simulink model "Model_Experiment2_LIFTEC_Paper_Ramon_version16a"  (R2020a)
settings: Solver=VariableStepAuto  StartTime=0.0  StopTime=6000  RelTol=1e-3
values from neighbouring files (symbols this model uses):
  k0_1 = x(1)    [Model_Calibration.m]
  k0_2 = x(2)    [Model_Calibration.m]
undefined symbols (not defined in the file or in its folder): alpha_1, alpha_2, Ccellini2, Ccellini3, Ccellini4, Ccellini5, Chini, Ctankini2, Ctankini3, Ctankini4, Ctankini5, d, D, E0, F, magnitude, N, R, r, S, T, Vcell, Vtank_Anolyte, Vtank_Catholyte
settings Model: Creator=Alejandro  LastModifiedBy=Alejandro
settings OptimizationCC: LifeSpan=inf
settings DebuggingCC: ArithmeticOperatorsInVariantConditions=warning
settings SFSimCC: CustomCodeUndefinedFunction=UseInterfaceOnly
settings CodeAppCC: StateflowObjectComments=on

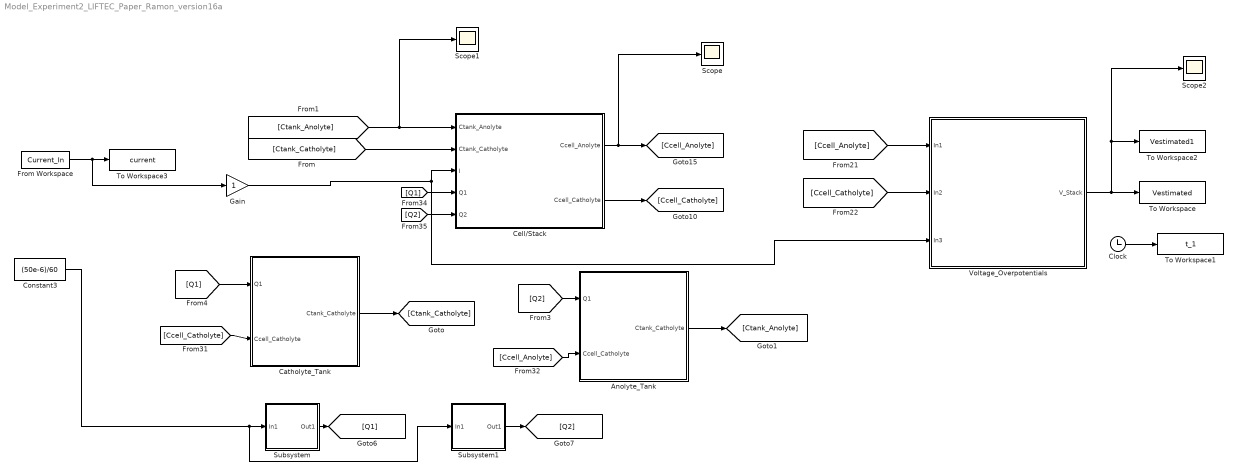
== system Model_Experiment2_LIFTEC_Paper_Ramon_version16a ==
  Anolyte_Tank : Subsystem  mask(Anolyte tank model){}
      mask help: This subsystem defines the model of the anolyte tank of the redox flow batteries..
      mask Help:
      | The parameters of the block consist on:
      | 
      | Vtank_Anolyte: Volume of the anolye tank (m^3)
      | Ctankini2: Initial concentration of V2 in the anolyte tank (mol/m^3)
      | Ctankini3: Initial concentration of V3 in the anolyte tank (mol/m^3)
      mask DialogControl Container4 Prompt: References
      mask DialogControl Control2 Prompt: 1] Tang, A.; McCann, J.; Bao, J.; Skyllas-Kazacos, M. Investigation of the effect of shunt current on battery efficiency and stack temperature in vanadium redox flow battery.
      mask DialogControl Control3 Prompt: https://doi.org/10.1016/j.jpowsour.2013.05.079.
      mask DialogControl Control4 Prompt: 2] Wei, Z.; Xiong, R.; Lim, T.M.; Meng, S.; Skyllas-Kazacos, M.  Online monitoring of state of charge and1010capacity loss for vanadium redox flow battery based on autoregressive exogenous modeling.
      mask DialogControl Control5 Prompt: https://doi.org/10.1016/j.jpowsour.2018.09.028.
      mask Display: image('Anolyte_Tank.JPG')
  Catholyte_Tank : Subsystem  mask(Catholyte tank model){}
      mask help: This subsystem defines the model of the catholyte tank of the redox flow batteries..
      mask Help:
      | The parameters of the block consist on:
      | 
      | Vtank_Catholyte: Volume of the catholyte tank (m^3)
      | Ctankini4: Initial concentration of V4 in the cell (mol/m^3)
      | Ctankini5: Initial concentration of V5 in the cell (mol/m^3)
      mask DialogControl Container4 Prompt: References
      mask DialogControl Control2 Prompt: 1] Tang, A.; McCann, J.; Bao, J.; Skyllas-Kazacos, M. Investigation of the effect of shunt current on battery efficiency and stack temperature in vanadium redox flow battery.
      mask DialogControl Control3 Prompt: https://doi.org/10.1016/j.jpowsour.2013.05.079.
      mask DialogControl Control4 Prompt: 2] Wei, Z.; Xiong, R.; Lim, T.M.; Meng, S.; Skyllas-Kazacos, M.  Online monitoring of state of charge and1010capacity loss for vanadium redox flow battery based on autoregressive exogenous modeling.
      mask DialogControl Control5 Prompt: https://doi.org/10.1016/j.jpowsour.2018.09.028.
      mask Display: image('Catholyte_Tank.JPG')
  Cell/Stack : Subsystem  mask(Cell-Stack model){}
      mask help: This subsystem defines the model of the cell or stack of the redox flow batteries.
      mask Help:
      | The parameters of the block consist on:
      | 
      | N: Number of cells
      | Vcell: Volume of a cell (m^3)
      | S: Electrode surface (m^2)
      | d: Thickness of the membrane (m)
      | Ccellini2: Initial concentration of V2 in the cell (mol/m^3)
      | Ccellini3: Initial concentration of V3 in the cell (mol/m^3)
      | Ccellini4: Initial concentration of V4 in the cell (mol/m^3)
      | Ccellini5: Initial concentration of V5 in the cell (mol/m^3)
      mask DialogControl Container7 Prompt: References
      mask DialogControl Control6 Prompt: 1] Tang, A.; McCann, J.; Bao, J.; Skyllas-Kazacos, M. Investigation of the effect of shunt current on battery efficiency and stack temperature in vanadium redox flow battery.
      mask DialogControl Control7 Prompt: 2] Wei, Z.; Xiong, R.; Lim, T.M.; Meng, S.; Skyllas-Kazacos, M.  Online monitoring of state of charge and1010capacity loss for vanadium redox flow battery based on autoregressive exogenous modeling.
      mask DialogControl Control8 Prompt: https://doi.org/10.1016/j.jpowsour.2018.09.028.
      mask Display: image('Cell.JPG')
  Clock : Clock
  Constant3 : Constant  Value=(50e-6)/60
  From Workspace : FromWorkspace  VariableName=Current_In
  Gain : Gain
  Scope : Scope
  Scope1 : Scope
  Scope2 : Scope
  Subsystem : Subsystem  mask(Pump model){Epump1=1}
      mask help: Model of the pump according to the manufacturer datasheet
      mask Help: Epump: Efficiency of the pump
      mask DialogControl Container4 Prompt: Manufacturer datasheet
      mask DialogControl Control2 Prompt: Model of the pump
      mask Display: image('Pump.JPG')
  Subsystem1 : Subsystem  mask(Pump model){Epump2=1}
      mask help: Model of the pump according to the manufacturer datasheet
      mask Help: Epump2 : Efficiency of the pump
      mask DialogControl Container4 Prompt: Manufacturer datasheet
      mask DialogControl Control2 Prompt: Model of the pump
      mask Display: image('Pump.JPG'); % Use "Edit Image" on toolstrip to change.
  To Workspace : ToWorkspace  VariableName=Vestimated  SampleTime=1.0187
      settings: Save2DSignal=2-D array (concatenate along first dimension)
  To Workspace1 : ToWorkspace  VariableName=t_1  SampleTime=1
      settings: Save2DSignal=2-D array (concatenate along first dimension)
  To Workspace2 : ToWorkspace  VariableName=Vestimated1  SampleTime=1
      settings: Save2DSignal=2-D array (concatenate along first dimension)
  To Workspace3 : ToWorkspace  VariableName=current  SampleTime=1.0
      settings: Save2DSignal=2-D array (concatenate along first dimension)
  Voltage_Overpotentials : Subsystem  mask(Voltage and overpotential){}
      mask help: This block computes the voltage and overpotentials of the cell-stack.
      mask Help:
      | The parameters of the block consist on:
      | 
      | E0: Standard electrode potential (V)
      | r: Ohmic resistance (Ohms)
      | Chini5: Initial concentration of H in the cell (mol/m^3)
      mask DialogControl Container3 Prompt: References
      mask DialogControl Control2 Prompt: (Add text here)
      mask DialogControl Control3 Prompt: (Add text here)
      mask Display: image('Voltage.png')
  wires:
  [Ccell_Catholyte] -> Voltage_Overpotentials/2(In2)
  [Q2] -> Anolyte_Tank/1(Q1)
  [Ccell_Anolyte] -> Anolyte_Tank/2(Ccell_Catholyte)
  [Q1] -> Cell/Stack/4(Q1)
  Catholyte_Tank/1(Ctank_Catholyte) -> [Ctank_Catholyte]
  [Ccell_Catholyte] -> Catholyte_Tank/2(Ccell_Catholyte)
  [Q2] -> Cell/Stack/5(Q2)
  Subsystem/1(Out1) -> [Q1]
  [Ctank_Anolyte] -> Scope1/1, Cell/Stack/1(Ctank_Anolyte)
  [Q1] -> Catholyte_Tank/1(Q1)
  [Ctank_Catholyte] -> Cell/Stack/2(Ctank_Catholyte)
  Subsystem1/1(Out1) -> [Q2]
  From Workspace/1 -> Gain/1, To Workspace3/1
  Constant3/1 -> Subsystem1/1(In1), Subsystem/1(In1)
  Cell/Stack/2(Ccell_Catholyte) -> [Ccell_Catholyte]
  Clock/1 -> To Workspace1/1
  Gain/1 -> Voltage_Overpotentials/3(In3), Cell/Stack/3("I ")
  [Ccell_Anolyte] -> Voltage_Overpotentials/1(In1)
  Anolyte_Tank/1(Ctank_Catholyte) -> [Ctank_Anolyte]
  Voltage_Overpotentials/1(V_Stack) -> Scope2/1, To Workspace2/1, To Workspace/1
  Cell/Stack/1(Ccell_Anolyte) -> Scope/1, [Ccell_Anolyte]

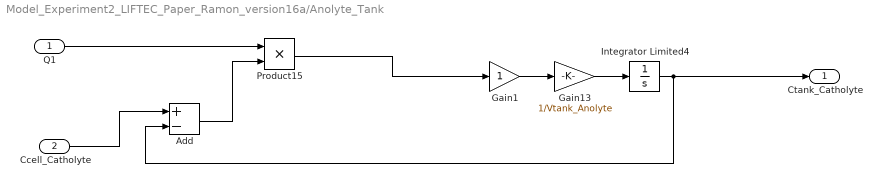
== system Model_Experiment2_LIFTEC_Paper_Ramon_version16a/Anolyte_Tank ==
  Q1 : Inport
  Ccell_Catholyte : Inport  Port=2
  Add : Sum  Inputs=+-
  Gain1 : Gain
  Gain13 : Gain  Gain=1/Vtank_Anolyte
  Integrator Limited4 : Integrator  InitialCondition=[Ctankini2 Ctankini3]  LimitOutput=on  UpperSaturationLimit=400  LowerSaturationLimit=0.001
  Product15 : Product
  Ctank_Catholyte : Outport
  wires:
  Gain13/1 -> Integrator Limited4/1
  Product15/1 -> Gain1/1
  Q1/1 -> Product15/1
  Integrator Limited4/1 -> Ctank_Catholyte/1, Add/2
  Gain1/1 -> Gain13/1
  Ccell_Catholyte/1 -> Add/1
  Add/1 -> Product15/2

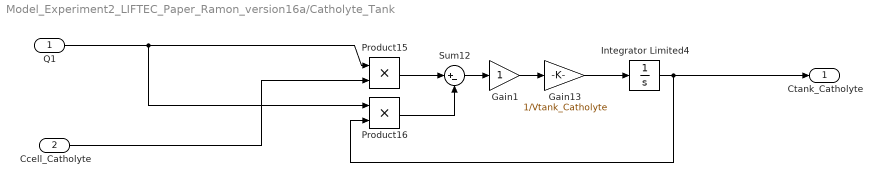
== system Model_Experiment2_LIFTEC_Paper_Ramon_version16a/Catholyte_Tank ==
  Q1 : Inport
  Ccell_Catholyte : Inport  Port=2
  Gain1 : Gain
  Gain13 : Gain  Gain=1/Vtank_Catholyte
  Integrator Limited4 : Integrator  InitialCondition=[Ctankini4 Ctankini5]  LimitOutput=on  UpperSaturationLimit=400  LowerSaturationLimit=0.001
  Product15 : Product
  Product16 : Product
  Sum12 : Sum  Inputs=|+-
  Ctank_Catholyte : Outport
  wires:
  Gain13/1 -> Integrator Limited4/1
  Sum12/1 -> Gain1/1
  Q1/1 -> Product16/1, Product15/1
  Integrator Limited4/1 -> Ctank_Catholyte/1, Product16/2
  Product15/1 -> Sum12/1
  Product16/1 -> Sum12/2
  Ccell_Catholyte/1 -> Product15/2
  Gain1/1 -> Gain13/1

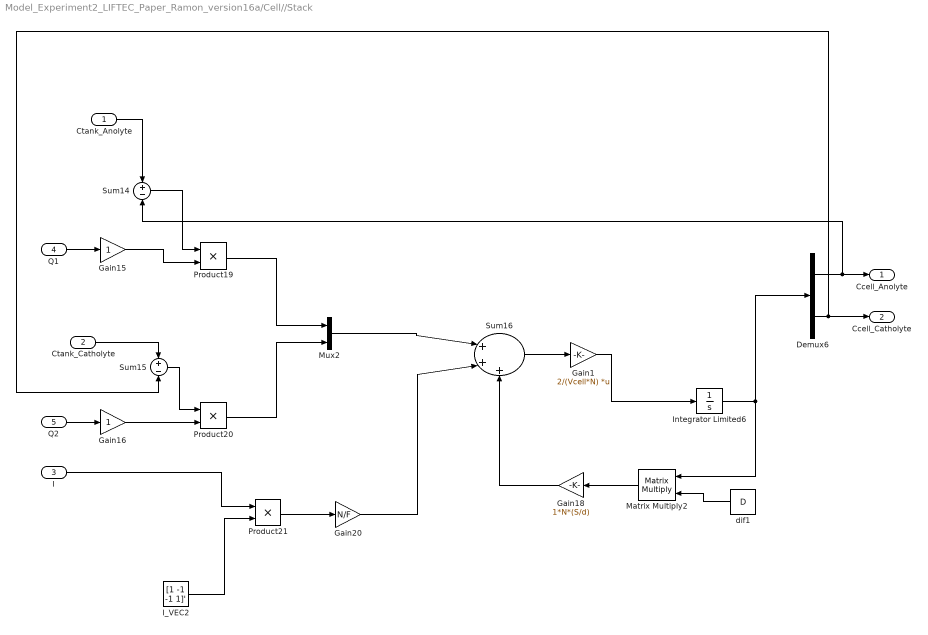
== system Model_Experiment2_LIFTEC_Paper_Ramon_version16a/Cell//Stack ==
  Ctank_Anolyte : Inport
  Ctank_Catholyte : Inport  Port=2
  "I " : Inport  Port=3
  Q1 : Inport  Port=4
  Q2 : Inport  Port=5
  Demux6 : Demux  Outputs=2
  Gain1 : Gain  Gain=2/(Vcell*N)  Multiplication=Matrix(K*u)
  Gain15 : Gain
  Gain16 : Gain
  Gain18 : Gain  Gain=1*N*(S/d)
  Gain20 : Gain  Gain=N/F
  I_VEC2 : Constant  Value=[1 -1 -1 1]'
  Integrator Limited6 : Integrator  InitialCondition=[Ccellini2 Ccellini3 Ccellini4 Ccellini5]  LimitOutput=on  UpperSaturationLimit=400  LowerSaturationLimit=0.001
  Matrix Multiply2 : Product  Multiplication=Matrix(*)
  Mux2 : Mux  Inputs=2
  Product19 : Product
  Product20 : Product
  Product21 : Product
  Sum14 : Sum  Inputs=+-
  Sum15 : Sum  Inputs=+-
  Sum16 : Sum  Inputs=|+++
  dif1 : Constant  Value=D
  Ccell_Anolyte : Outport
  Ccell_Catholyte : Outport  Port=2
  wires:
  Gain18/1 -> Sum16/3
  Ctank_Anolyte/1 -> Sum14/1
  Gain20/1 -> Sum16/2
  "I "/1 -> Product21/1
  Integrator Limited6/1 -> Matrix Multiply2/1, Demux6/1
  Sum16/1 -> Gain1/1
  Gain15/1 -> Product19/2
  Sum14/1 -> Product19/1
  Product21/1 -> Gain20/1
  I_VEC2/1 -> Product21/2
  Product19/1 -> Mux2/1
  Sum15/1 -> Product20/1
  Gain16/1 -> Product20/2
  Q1/1 -> Gain15/1
  Matrix Multiply2/1 -> Gain18/1
  dif1/1 -> Matrix Multiply2/2
  Product20/1 -> Mux2/2
  Ctank_Catholyte/1 -> Sum15/1
  Q2/1 -> Gain16/1
  Mux2/1 -> Sum16/1
  Gain1/1 -> Integrator Limited6/1
  Demux6/1 -> Sum14/2, Ccell_Anolyte/1
  Demux6/2 -> Ccell_Catholyte/1, Sum15/2

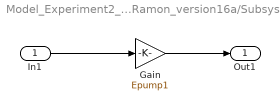
== system Model_Experiment2_LIFTEC_Paper_Ramon_version16a/Subsystem ==
  In1 : Inport
  Gain : Gain  Gain=Epump1
  Out1 : Outport
  wires:
  In1/1 -> Gain/1
  Gain/1 -> Out1/1

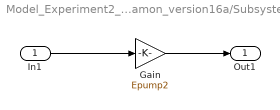
== system Model_Experiment2_LIFTEC_Paper_Ramon_version16a/Subsystem1 ==
  In1 : Inport
  Gain : Gain  Gain=Epump2
  Out1 : Outport
  wires:
  In1/1 -> Gain/1
  Gain/1 -> Out1/1

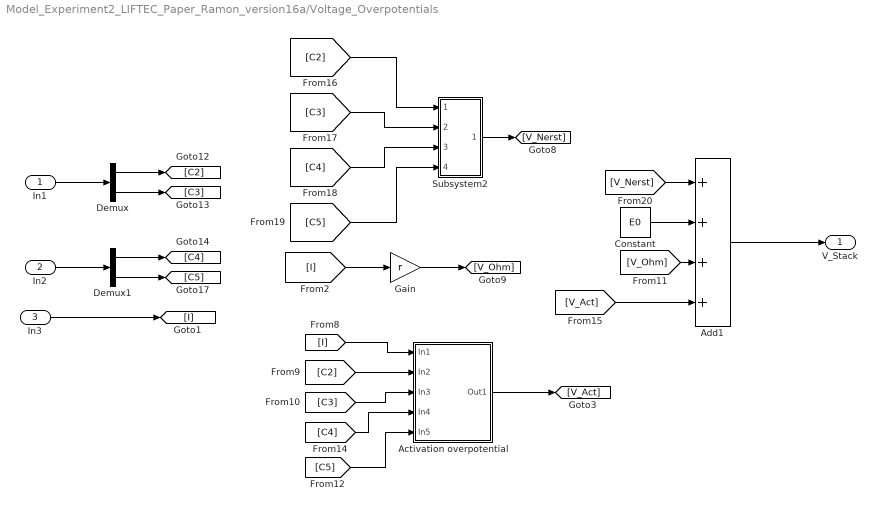
== system Model_Experiment2_LIFTEC_Paper_Ramon_version16a/Voltage_Overpotentials ==
  In1 : Inport
  In2 : Inport  Port=2
  In3 : Inport  Port=3
  Activation overpotential : Subsystem
  Add1 : Sum  Inputs=++++
  Constant : Constant  Value=E0
  Demux : Demux  Outputs=2
  Demux1 : Demux  Outputs=2
  Gain : Gain  Gain=r
  Subsystem2 : Subsystem
  V_Stack : Outport
  wires:
  Add1/1 -> V_Stack/1
  Demux/2 -> [C3]
  Subsystem2/1(Out1) -> [V_Nerst]
  Demux1/2 -> [C5]
  Demux1/1 -> [C4]
  [V_Nerst] -> Add1/1
  Constant/1 -> Add1/2
  Demux/1 -> [C2]
  [V_Ohm] -> Add1/3
  [C2] -> Subsystem2/1(In1)
  [C5] -> Subsystem2/4(In4)
  [C3] -> Subsystem2/2(In2)
  [C4] -> Subsystem2/3(In3)
  In1/1 -> Demux/1
  In2/1 -> Demux1/1
  In3/1 -> [I]
  Gain/1 -> [V_Ohm]
  [I] -> Gain/1
  [I] -> Activation overpotential/1(In1)
  [C2] -> Activation overpotential/2(In2)
  [C3] -> Activation overpotential/3(In3)
  [C4] -> Activation overpotential/4(In4)
  [C5] -> Activation overpotential/5(In5)
  Activation overpotential/1(Out1) -> [V_Act]
  [V_Act] -> Add1/4

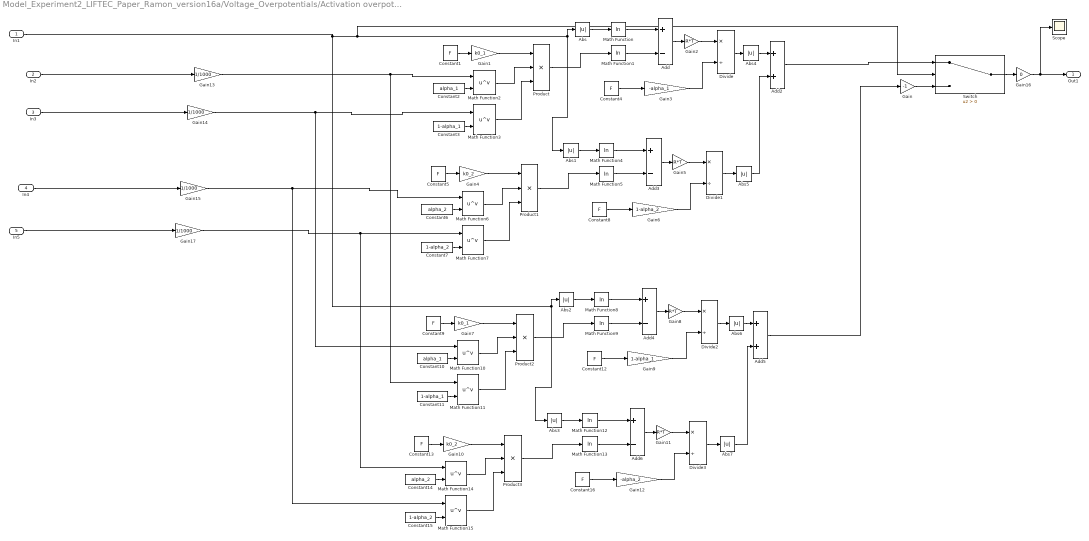
== system Model_Experiment2_LIFTEC_Paper_Ramon_version16a/Voltage_Overpotentials/Activation overpotential ==
  In1 : Inport
  In2 : Inport  Port=2
  In3 : Inport  Port=3
  In4 : Inport  Port=4
  In5 : Inport  Port=5
  Abs{,1..7} (8 alike) : Abs
  Add{,3..4,6} (4 alike) : Sum  Inputs=+-
  Add2 : Sum
  Add5 : Sum
  Constant{1,4..5,8..9,12..13,16} (8 alike) : Constant  Value=F
  Constant10 : Constant  Value=alpha_1
  Constant11 : Constant  Value=1-alpha_1
  Constant14 : Constant  Value=alpha_2
  Constant15 : Constant  Value=1-alpha_2
  Constant2 : Constant  Value=alpha_1
  Constant3 : Constant  Value=1-alpha_1
  Constant6 : Constant  Value=alpha_2
  Constant7 : Constant  Value=1-alpha_2
  Divide{,1..3} (4 alike) : Product  Inputs=*/
  Gain : Gain  Gain=-1
  Gain1 : Gain  Gain=k0_1
  Gain10 : Gain  Gain=k0_2
  Gain{2,5,8,11} (4 alike) : Gain  Gain=R*T
  Gain12 : Gain  Gain=-alpha_2
  Gain{13..15,17} (4 alike) : Gain  Gain=1/1000
  Gain16 : Gain  Gain=0
  Gain3 : Gain  Gain=-alpha_1
  Gain4 : Gain  Gain=k0_2
  Gain6 : Gain  Gain=1-alpha_2
  Gain7 : Gain  Gain=k0_1
  Gain9 : Gain  Gain=1-alpha_1
  Math Function{,1,4..5,8..9,12..13} (8 alike) : Math  Operator=log  SignedPower=on  SaturateOnIntegerOverflow=on
  Math Function{2..3,6..7,10..11,14..15} (8 alike) : Math  Operator=pow  SignedPower=on  SaturateOnIntegerOverflow=on
  Product{,1..3} (4 alike) : Product  Inputs=3
  Scope : Scope
  Switch : Switch  Criteria=u2 > Threshold
  Out1 : Outport
  wires:
  Divide/1 -> Abs4/1
  Constant1/1 -> Gain1/1
  Constant5/1 -> Gain4/1
  In5/1 -> Gain17/1
  Product1/1 -> Math Function5/1
  In1/1 -> Abs2/1, Abs3/1, Switch/2, Abs/1, Abs1/1
  Abs/1 -> Math Function/1
  Constant8/1 -> Gain6/1
  Constant2/1 -> Math Function2/2
  Math Function2/1 -> Product/2
  Gain5/1 -> Divide1/1
  Math Function5/1 -> Add3/2
  Add/1 -> Gain2/1
  Math Function4/1 -> Add3/1
  Gain12/1 -> Divide3/2
  Add6/1 -> Gain11/1
  Switch/1 -> Gain16/1
  Constant7/1 -> Math Function7/2
  Constant15/1 -> Math Function15/2
  Gain3/1 -> Divide/2
  Abs1/1 -> Math Function4/1
  Product3/1 -> Math Function13/1
  Add4/1 -> Gain8/1
  Math Function7/1 -> Product1/3
  In4/1 -> Gain15/1
  Constant3/1 -> Math Function3/2
  Product2/1 -> Math Function9/1
  Gain6/1 -> Divide1/2
  Gain8/1 -> Divide2/1
  Math Function6/1 -> Product1/2
  Constant14/1 -> Math Function14/2
  Gain4/1 -> Product1/1
  Constant6/1 -> Math Function6/2
  In3/1 -> Gain14/1
  Gain1/1 -> Product/1
  Math Function15/1 -> Product3/3
  Constant13/1 -> Gain10/1
  Gain11/1 -> Divide3/1
  Gain10/1 -> Product3/1
  Constant11/1 -> Math Function11/2
  Abs2/1 -> Math Function8/1
  Math Function8/1 -> Add4/1
  Product/1 -> Math Function1/1
  Constant12/1 -> Gain9/1
  Divide1/1 -> Abs5/1
  Math Function3/1 -> Product/3
  Gain9/1 -> Divide2/2
  Divide2/1 -> Abs6/1
  Gain7/1 -> Product2/1
  Gain2/1 -> Divide/1
  Constant4/1 -> Gain3/1
  Divide3/1 -> Abs7/1
  Math Function11/1 -> Product2/3
  Add3/1 -> Gain5/1
  Add5/1 -> Gain/1
  Abs3/1 -> Math Function12/1
  Constant10/1 -> Math Function10/2
  Math Function9/1 -> Add4/2
  Math Function14/1 -> Product3/2
  Math Function10/1 -> Product2/2
  Math Function13/1 -> Add6/2
  Math Function12/1 -> Add6/1
  Constant16/1 -> Gain12/1
  Constant9/1 -> Gain7/1
  In2/1 -> Gain13/1
  Math Function/1 -> Add/1
  Math Function1/1 -> Add/2
  Gain13/1 -> Math Function11/1, Math Function2/1
  Gain14/1 -> Math Function10/1, Math Function3/1
  Gain15/1 -> Math Function15/1, Math Function6/1
  Gain17/1 -> Math Function14/1, Math Function7/1
  Gain/1 -> Switch/3
  Add2/1 -> Switch/1
  Abs4/1 -> Add2/1
  Abs5/1 -> Add2/2
  Abs6/1 -> Add5/1
  Abs7/1 -> Add5/2
  Gain16/1 -> Scope/1, Out1/1

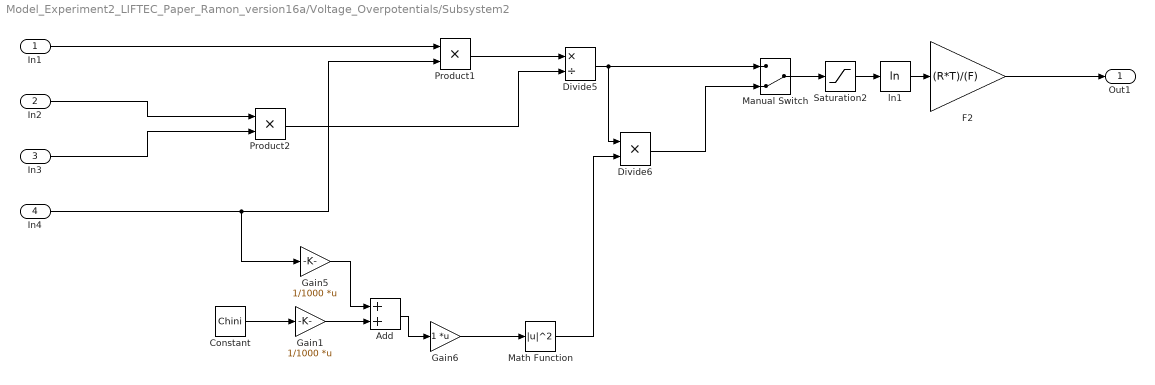
== system Model_Experiment2_LIFTEC_Paper_Ramon_version16a/Voltage_Overpotentials/Subsystem2 ==
  In1 : Inport
  In2 : Inport  Port=2
  In3 : Inport  Port=3
  In4 : Inport  Port=4
  Add : Sum
  Constant : Constant  Value=Chini
  Divide5 : Product  Inputs=*/
  Divide6 : Product  Inputs=**
  F2 : Gain  Gain=(R*T)/(F)
  Gain1 : Gain  Gain=1/1000  Multiplication=Matrix(K*u)
  Gain5 : Gain  Gain=1/1000  Multiplication=Matrix(K*u)
  Gain6 : Gain  Multiplication=Matrix(K*u)
  Manual Switch : ManualSwitch  CurrentSetting=0
  Math Function : Math  Operator=magnitude^2  SignedPower=on  SaturateOnIntegerOverflow=on
  Product1 : Product
  Product2 : Product
  Saturation2 : Saturate  UpperLimit=1e5  LowerLimit=1e-5
  ln1 : Math  Operator=log  SignedPower=on  SaturateOnIntegerOverflow=on
  Out1 : Outport
  wires:
  Gain5/1 -> Add/1
  Gain6/1 -> Math Function/1
  Manual Switch/1 -> Saturation2/1
  Product1/1 -> Divide5/1
  In3/1 -> Product2/2
  ln1/1 -> F2/1
  Divide6/1 -> Manual Switch/2
  Add/1 -> Gain6/1
  Divide5/1 -> Divide6/1, Manual Switch/1
  Constant/1 -> Gain1/1
  Saturation2/1 -> ln1/1
  In2/1 -> Product2/1
  In4/1 -> Gain5/1, Product1/2
  Math Function/1 -> Divide6/2
  Product2/1 -> Divide5/2
  F2/1 -> Out1/1
  In1/1 -> Product1/1
  Gain1/1 -> Add/2
